simulink model "HWq3"  (R2025a)
settings: Solver=VariableStepAuto  StartTime=0.0  StopTime=0.001  MaxStep=0.00000002  MinStep=0.00000001  RelTol=1e-3
libraries: spsVoltageMeasurementLib x5, spsIdealSwitchLib x4, spsSeriesRLCBranchLib x3, spsDiodeLib x2, spsDCVoltageSourceLib x1, spsMultiWindingTransformerLib x1, simulink x1, spsCurrentMeasurementLib x1, spspowerguiLib x1
settings Model: Creator=kerim  LastModifiedBy=kerim
settings SolverCC: InitialStep=0.00000001
settings DataIOCC: InitialState=out.xFinal  SaveFormat=Array

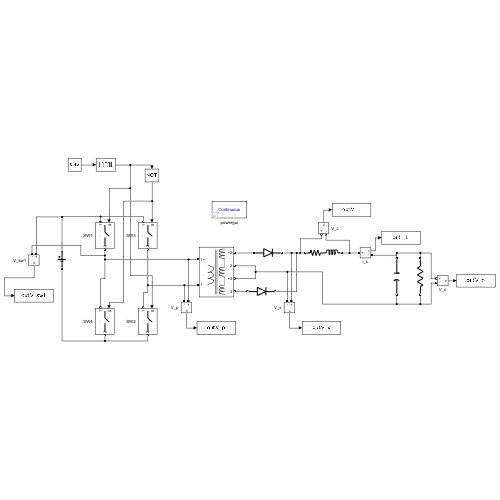
[thumbnail: Simulink's stored preview of the top-level diagram]
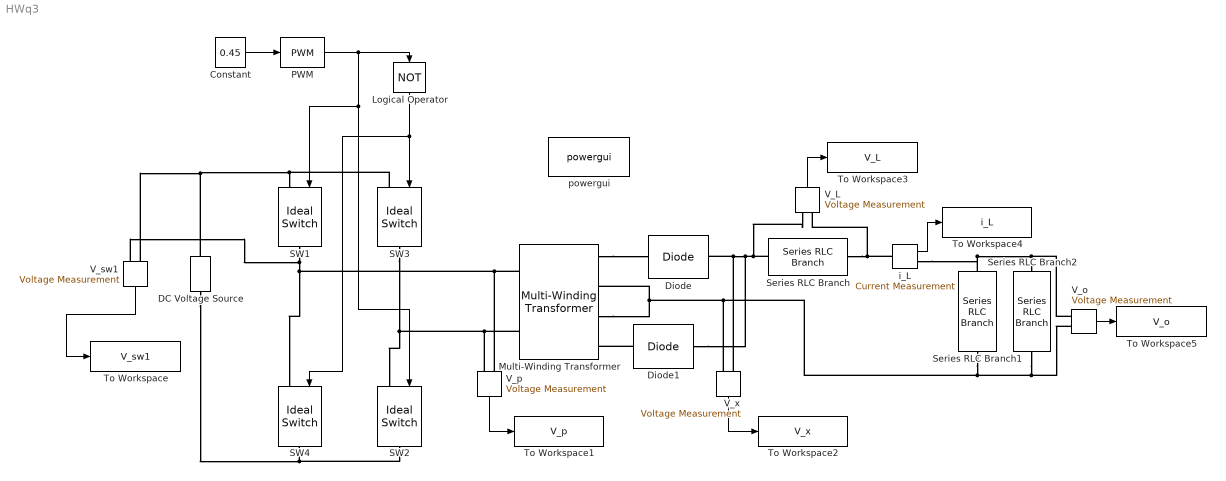
== system HWq3 ==
  Constant : Constant  Value=0.45
  DC Voltage Source : spsDCVoltageSourceLib/DC Voltage Source  Amplitude=100  Measurements=None
  Diode : spsDiodeLib/Diode  Ron=0  Lon=0  Vf=0  IC=0  UseSnubber=0  Rs=0  Cs=0  Measurements=off
  Diode1 : spsDiodeLib/Diode  Ron=0  Lon=0  Vf=0  IC=0  UseSnubber=0  Rs=0  Cs=0  Measurements=off
  Logical Operator : Logic  Operator=NOT  AllPortsSameDT=off  OutDataTypeStr=boolean
  Multi-Winding Transformer : spsMultiWindingTransformerLib/Multi-Winding Transformer  LeftWindings=1  RightWindings=2  TappedWindings=no taps  NumberOfTaps=2  SetSaturation=off  Hysteresis=off  DataFile='hysteresis.mat'  Measurements=None  UNITS=SI  NominalPower=[250 50]  NominalVoltages="[100  26.667  26.667]"  WindingResistances=[0.0411 0.00334 0.00334]  WindingInductances=[0 0 0]  Rm=Inf  Lm=0.00106  Saturation=[0 0;0.0084853 0.54019;3.5355 0.68424]  SpecifyInitialFlux=off  InitialFlux=0  BreakLoop=off  DiscreteSolver=Trapezoidal iterative  DataType=on  TransfoNumber=1
      settings: LibrarySourceBlock=|
      | sps_lib/Power Grid Elements/Multi-Winding
      | Transformer
  PWM : simulink/Discontinuities/PWM  DisableCoverage=on  Period=1/(200e3)  InitialDelay=0  DisallowZeroDutyCycle=off  RunAtFixedTimeIntervals=off  SampleTime=0.1
  SW{1..4} (4 alike) : spsIdealSwitchLib/Ideal Switch  Ron=0  Lon=0  IC=0  Rs=0  Cs=0  Measurements=off
  Series RLC Branch : spsSeriesRLCBranchLib/Series RLC Branch  LConnTagsString=__new0  RConnTagsString=__new0  BranchType=RL  Resistance=2.96*10^-3  Inductance=5.96*10^-6  SetiL0=off  InitialCurrent=0  Capacitance=1e-6  Setx0=off  InitialVoltage=0  Measurements=None
  Series RLC Branch1 : spsSeriesRLCBranchLib/Series RLC Branch  LConnTagsString=__new0  RConnTagsString=__new0  BranchType=C  Resistance=1  Inductance=1e-3  SetiL0=off  InitialCurrent=0  Capacitance=1.36*10^-6  Setx0=off  InitialVoltage=0  Measurements=None
  Series RLC Branch2 : spsSeriesRLCBranchLib/Series RLC Branch  LConnTagsString=__new0  RConnTagsString=__new0  BranchType=R  Resistance=2.304  Inductance=1e-3  SetiL0=off  InitialCurrent=0  Capacitance=1e-6  Setx0=off  InitialVoltage=0  Measurements=None
  To Workspace : ToWorkspace  VariableName=V_sw1  SampleTime=-1
  To Workspace1 : ToWorkspace  VariableName=V_p  SampleTime=-1
  To Workspace2 : ToWorkspace  VariableName=V_x  SampleTime=-1
  To Workspace3 : ToWorkspace  VariableName=V_L  SampleTime=-1
  To Workspace4 : ToWorkspace  VariableName=i_L  SampleTime=-1
  To Workspace5 : ToWorkspace  VariableName=V_o  SampleTime=-1
  V_L : spsVoltageMeasurementLib/Voltage Measurement  PhasorSimulation=off  OutputType=Complex  PSBequivalent=0
  V_o : spsVoltageMeasurementLib/Voltage Measurement  PhasorSimulation=off  OutputType=Complex  PSBequivalent=0
  V_p : spsVoltageMeasurementLib/Voltage Measurement  PhasorSimulation=off  OutputType=Complex  PSBequivalent=0
  V_sw1 : spsVoltageMeasurementLib/Voltage Measurement  PhasorSimulation=off  OutputType=Complex  PSBequivalent=0
  V_x : spsVoltageMeasurementLib/Voltage Measurement  PhasorSimulation=off  OutputType=Complex  PSBequivalent=0
  i_L : spsCurrentMeasurementLib/Current Measurement  PhasorSimulation=off  OutputType=Complex  PSBequivalent=0
  powergui : spspowerguiLib/powergui  Priority=1  SimulationMode=Continuous  SampleTime=50e-6  frequency=60  Iterations=50  frequencyindice=0  Pbase=100e6  ErrMax=1e-4  UnitsV=kV  UnitsW=MW  buscounter=0  FunctionMessages=off  echomessages=off  EnableUseOfTLC=off  CurrentSourceSwitches=off  DisableSnubberDevices=off  DisableRonSwitches=off  DisableVfSwitches=off  DisplayEquations=off  AutomaticDiscreteSolvers=off  SolverType=Tustin/Backward Euler (TBE)  Interpol=off  ExternalGateDelay=off  methode=off  Ts=100  x0status=blocks  SPID=on  SwTol=0  HookPort=off  NonlinearTolerance=1e-4  nMaxIteration=100  ContinueOnMaxIteration=off  RestoreLinks=warning  ResistiveCurrentMeasurement=off  Frange=[0:2:500]  Ylog=off  Xlog=on  ShowGrid=off  save=off  variable=ZData  structure=0  ZoomFFT=off  StartTime=0.0  cycles=1  DisplayStyle=1  fundamental=60  FreqAxis=off  MaxFrequency=1000  frequencyindicesteady=1  RmsSteady=1  display=off
  wires:
  Constant/1 -> PWM/1
  Logical Operator/1 -> SW4/1, SW3/1
  PWM/1 -> SW1/1, SW2/1, Logical Operator/1
  V_sw1/1 -> To Workspace/1
  V_p/1 -> To Workspace1/1
  V_x/1 -> To Workspace2/1
  V_L/1 -> To Workspace3/1
  i_L/1 -> To Workspace4/1
  V_o/1 -> To Workspace5/1
  connections:
  DC Voltage Source/RConn1 -- V_sw1/LConn1 -- SW3/LConn1 -- SW1/LConn1
  DC Voltage Source/LConn1 -- SW2/RConn1 -- SW4/RConn1
  SW1/RConn1 -- V_sw1/LConn2 -- V_p/LConn1 -- Multi-Winding Transformer/LConn1 -- SW4/LConn1
  SW3/RConn1 -- V_p/LConn2 -- Multi-Winding Transformer/LConn2 -- SW2/LConn1
  Diode1/LConn1 -- Multi-Winding Transformer/RConn4
  Multi-Winding Transformer/RConn1 -- Diode/LConn1
  Multi-Winding Transformer/RConn3 -- Series RLC Branch2/RConn1 -- V_o/LConn2 -- Series RLC Branch1/RConn1 -- V_x/LConn2 -- Multi-Winding Transformer/RConn2
  Series RLC Branch/LConn1 -- V_L/LConn1 -- V_x/LConn1 -- Diode/RConn1 -- Diode1/RConn1
  Series RLC Branch1/LConn1 -- i_L/RConn1 -- V_o/LConn1 -- Series RLC Branch2/LConn1
  Series RLC Branch/RConn1 -- i_L/LConn1 -- V_L/LConn2
